simulink model "Crazyflie_NoLinealModel"  (R2020b)
settings: Solver=FixedStepAuto  StartTime=0.0  StopTime=30  FixedStep=0.01  RelTol=1e-3
values from neighbouring files (symbols this model uses):
  fm = 0.2685    [Crazyflie_Model.m]
  g = 9.81    [Crazyflie_Model.m]
  Ixx = 1.395e-05    [Crazyflie_Model.m]
  Iyy = 1.395e-05    [Crazyflie_Model.m]
  Izz = 2.173e-05    [Crazyflie_Model.m]
  m = 0.027    [Crazyflie_Model.m]
  MNL1 = [         CT,           CT,           CT,           CT ... (first row only)    [Crazyflie_Model.m]
  we = sqrt((m*g)/(4*CT))    [Crazyflie_Model.m]
undefined symbols (not defined in the file or in its folder): fs_outer, KDp, KDphi, KDq, KDr, KDtheta, KDxp, KDxv, KDy, KDyaw, KDz, KIp, KIphi, KIq, KIr, KItheta, KIxp, KIxv, KIy, KIyaw, KIz, KPp, KPphi, KPq, KPr, KPtheta, KPxp, KPxv, KPy, KPyaw, KPz, MCO, phi_theta_limit, xyv_lim
libraries: pid_lib x11, simulink x2
settings Model: Creator=Rafael  LastModifiedBy=FranciscoJose
settings DataIOCC: LimitDataPoints=on  SaveFormat=Array  SignalLoggingSaveFormat=ModelDataLogs  ReturnWorkspaceOutputs=off
settings OptimizationCC: ExpressionDepthLimit=2147483647  LifeSpan=inf
settings DebuggingCC: UnderspecifiedInitializationDetection=Classic  MergeDetectMultiDrivingBlocksExec=none  SolverPrmCheckMsg=warning  FcnCallInpInsideContextMsg=warning  AllowSymbolicDim=off  StateNameClashWarn=warning  SFUnexpectedBacktrackingDiag=warning  SFNoUnconditionalDefaultTransitionDiag=warning  SFExecutionAtInitializationDiag=none  ArithmeticOperatorsInVariantConditions=warning
settings HardwareCC: ProdBitPerPointer=32  ProdBitPerSizeT=32  ProdBitPerPtrDiffT=32  ProdLargestAtomicFloat=None  ProdIntDivRoundTo=Undefined  ProdEndianess=Unspecified  ProdWordSize=32  ProdHWDeviceType=32-bit Generic
settings ModelReferenceCC: PropagateSignalLabelsOutOfModel=off
settings SFSimCC: SimUseLocalCustomCode=off  CustomCodeUndefinedFunction=UseInterfaceOnly
settings RTWCC: RTWUseLocalCustomCode=off
settings CodeAppCC: StateflowObjectComments=on
settings GRTTargetCC: TargetLangStandard=C89/C90 (ANSI)
settings ConfigComp: CovMetricSettings=dw  CovSaveCumulativeToWorkspaceVar=on  CovSaveSingleToWorkspaceVar=on  CovExternalEMLEnable=off
settings SimscapeCC: SimscapeNormalizeSystem=off
settings ConfigurationSet: Description=SimMechanics 2G

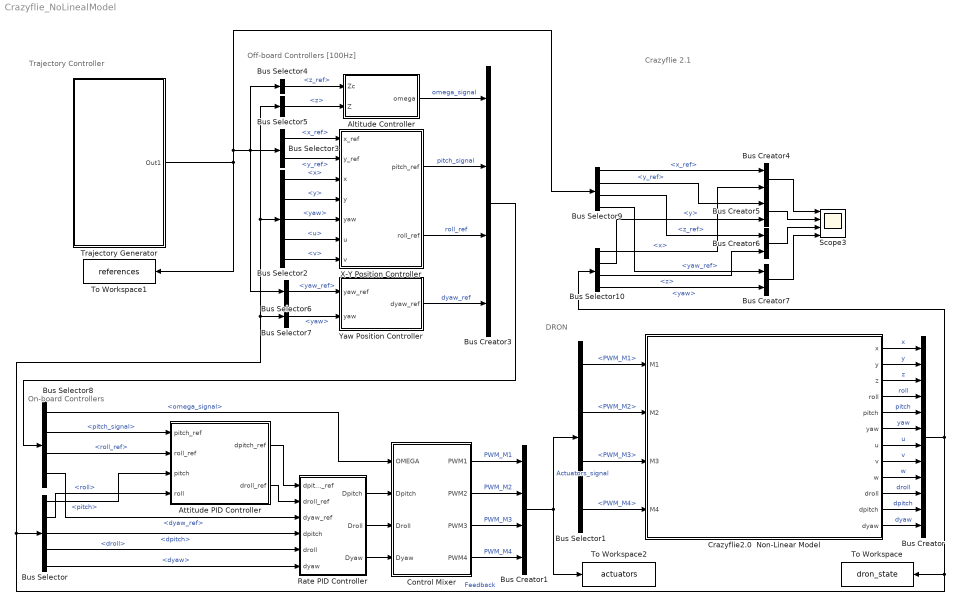
== system Crazyflie_NoLinealModel ==
  note: DRON
  note: Trajectory Controller
  note: Off-board Controllers [100Hz]
  note: On-board Controllers
  note: Crazyflie 2.1
  Altitude Controller : Subsystem
  Attitude PID Controller : Subsystem
  Bus Creator : BusCreator  Inputs=12
  Bus Creator1 : BusCreator  Inputs=4
  Bus Creator3 : BusCreator  Inputs=4
  Bus Creator{4..7} (4 alike) : BusCreator  Inputs=2
  Bus Selector : BusSelector  OutputSignals=pitch,roll,dpitch,droll,dyaw
  Bus Selector1 : BusSelector  OutputSignals=PWM_M1,PWM_M2,PWM_M3,PWM_M4
  Bus Selector10 : BusSelector  OutputSignals=x,y,z,yaw
  Bus Selector2 : BusSelector  OutputSignals=x,y,yaw,u,v
  Bus Selector3 : BusSelector  OutputSignals=x_ref,y_ref
  Bus Selector4 : BusSelector  OutputSignals=z_ref
  Bus Selector5 : BusSelector  OutputSignals=z
  Bus Selector6 : BusSelector  OutputSignals=yaw_ref
  Bus Selector7 : BusSelector  OutputSignals=yaw
  Bus Selector8 : BusSelector  OutputSignals=omega_signal,pitch_signal,roll_ref,dyaw_ref
  Bus Selector9 : BusSelector  OutputSignals=x_ref,y_ref,z_ref,yaw_ref
  Control Mixer : Subsystem
  Crazyflie2.0  Non-Linear Model : Subsystem
      mask Display: image('$imagefile'); % Use "Edit Image" on toolstrip to change.
  Rate PID Controller : Subsystem
  Scope3 : Scope  NumInputPorts=4
  To Workspace : ToWorkspace  VariableName=dron_state  SaveFormat=Timeseries  SampleTime=-1
  To Workspace1 : ToWorkspace  VariableName=references  SaveFormat=Timeseries  SampleTime=-1
  To Workspace2 : ToWorkspace  VariableName=actuators  SaveFormat=Timeseries  SampleTime=-1
  Trajectory Generator : Subsystem
  X-Y Position Controller : Subsystem
  Yaw Position Controller : Subsystem
  wires:
  Crazyflie2.0  Non-Linear Model/11(dpitch) -> Bus Creator/11  "dpitch"
  Crazyflie2.0  Non-Linear Model/3(z) -> Bus Creator/3  "z"
  Crazyflie2.0  Non-Linear Model/12(dyaw) -> Bus Creator/12  "dyaw"
  Crazyflie2.0  Non-Linear Model/4(roll) -> Bus Creator/4  "roll"
  Crazyflie2.0  Non-Linear Model/5(pitch) -> Bus Creator/5  "pitch"
  Crazyflie2.0  Non-Linear Model/6(yaw) -> Bus Creator/6  "yaw"
  Crazyflie2.0  Non-Linear Model/1(x) -> Bus Creator/1  "x"
  Crazyflie2.0  Non-Linear Model/2(y) -> Bus Creator/2  "y"
  Crazyflie2.0  Non-Linear Model/7(u) -> Bus Creator/7  "u"
  Crazyflie2.0  Non-Linear Model/8(v) -> Bus Creator/8  "v"
  Crazyflie2.0  Non-Linear Model/9(w) -> Bus Creator/9  "w"
  Crazyflie2.0  Non-Linear Model/10(droll) -> Bus Creator/10  "droll"
  Bus Creator/1 -> Bus Selector10/1, Bus Selector/1, Bus Selector5/1, Bus Selector2/1, Bus Selector7/1, To Workspace/1  "Feedback"
  Bus Selector/5 -> Rate PID Controller/6(dyaw)  "<dyaw>"
  Control Mixer/1(PWM1) -> Bus Creator1/1  "PWM_M1"
  Control Mixer/2(PWM2) -> Bus Creator1/2  "PWM_M2"
  Control Mixer/3(PWM3) -> Bus Creator1/3  "PWM_M3"
  Control Mixer/4(PWM4) -> Bus Creator1/4  "PWM_M4"
  Bus Creator1/1 -> Bus Selector1/1, To Workspace2/1  "Actuators_signal"
  Bus Selector1/1 -> Crazyflie2.0  Non-Linear Model/1(M1)  "<PWM_M1>"
  Bus Selector1/2 -> Crazyflie2.0  Non-Linear Model/2(M2)  "<PWM_M2>"
  Bus Selector1/3 -> Crazyflie2.0  Non-Linear Model/3(M3)  "<PWM_M3>"
  Bus Selector1/4 -> Crazyflie2.0  Non-Linear Model/4(M4)  "<PWM_M4>"
  Bus Selector4/1 -> Altitude Controller/1(Zc)  "<z_ref>"
  Altitude Controller/1(omega) -> Bus Creator3/1  "omega_signal"
  Bus Selector3/1 -> X-Y Position Controller/1(x_ref)  "<x_ref>"
  Bus Selector3/2 -> X-Y Position Controller/2(y_ref)  "<y_ref>"
  Bus Selector2/1 -> X-Y Position Controller/3(x)  "<x>"
  Bus Selector2/2 -> X-Y Position Controller/4(y)  "<y>"
  Bus Selector2/3 -> X-Y Position Controller/5(yaw)  "<yaw>"
  Bus Selector2/4 -> X-Y Position Controller/6(u)  "<u>"
  Bus Selector2/5 -> X-Y Position Controller/7(v)  "<v>"
  X-Y Position Controller/1(pitch_ref) -> Bus Creator3/2  "pitch_signal"
  X-Y Position Controller/2(roll_ref) -> Bus Creator3/3  "roll_ref"
  Bus Selector5/1 -> Altitude Controller/2(Z)  "<z>"
  Bus Selector6/1 -> Yaw Position Controller/1(yaw_ref)  "<yaw_ref>"
  Bus Selector7/1 -> Yaw Position Controller/2(yaw)  "<yaw>"
  Yaw Position Controller/1(dyaw_ref) -> Bus Creator3/4  "dyaw_ref"
  Bus Creator3/1 -> Bus Selector8/1
  Bus Selector8/1 -> Control Mixer/1(OMEGA)  "<omega_signal>"
  Bus Selector8/2 -> Attitude PID Controller/1(pitch_ref)  "<pitch_signal>"
  Bus Selector8/3 -> Attitude PID Controller/2(roll_ref)  "<roll_ref>"
  Bus Selector8/4 -> Rate PID Controller/3(dyaw_ref)  "<dyaw_ref>"
  Rate PID Controller/1(Dpitch) -> Control Mixer/2(Dpitch)
  Rate PID Controller/3(Dyaw) -> Control Mixer/4(Dyaw)
  Bus Creator4/1 -> Scope3/1
  Bus Creator5/1 -> Scope3/2
  Bus Creator6/1 -> Scope3/3
  Bus Creator7/1 -> Scope3/4
  Bus Selector9/1 -> Bus Creator4/1  "<x_ref>"
  Bus Selector9/2 -> Bus Creator5/1  "<y_ref>"
  Bus Selector9/3 -> Bus Creator6/1  "<z_ref>"
  Bus Selector9/4 -> Bus Creator7/1  "<yaw_ref>"
  Bus Selector10/1 -> Bus Creator4/2  "<x>"
  Bus Selector10/2 -> Bus Creator5/2  "<y>"
  Bus Selector10/3 -> Bus Creator6/2  "<z>"
  Bus Selector10/4 -> Bus Creator7/2  "<yaw>"
  Rate PID Controller/2(Droll) -> Control Mixer/3(Droll)
  Attitude PID Controller/1(dpitch_ref) -> Rate PID Controller/1(dpitch_ref)
  Attitude PID Controller/2(droll_ref) -> Rate PID Controller/2(droll_ref)
  Bus Selector/1 -> Attitude PID Controller/3(pitch)  "<pitch>"
  Bus Selector/2 -> Attitude PID Controller/4(roll)  "<roll>"
  Bus Selector/3 -> Rate PID Controller/4(dpitch)  "<dpitch>"
  Bus Selector/4 -> Rate PID Controller/5(droll)  "<droll>"
  Trajectory Generator/1(Out1) -> To Workspace1/1, Bus Selector9/1, Bus Selector6/1, Bus Selector4/1, Bus Selector3/1

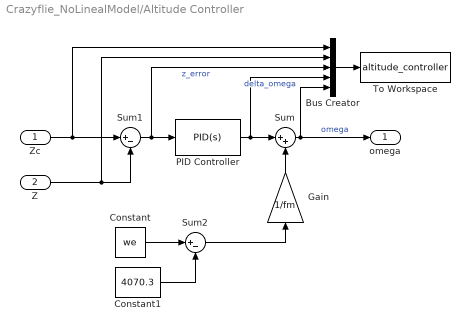
== system Crazyflie_NoLinealModel/Altitude Controller ==
  Zc : Inport
  Z : Inport  Port=2
  Bus Creator : BusCreator  Inputs=5
  Constant : Constant  Value=we
  Constant1 : Constant  Value=4070.3
  Gain : Gain  Gain=1/fm
  PID Controller : pid_lib/PID Controller  Controller=PID  Form=Parallel  TimeDomain=Continuous-time  UseExternalTs=off  SampleTime=-1  IntegratorMethod=Forward Euler  FilterMethod=Forward Euler  ControllerParametersSource=internal  P=KPz  I=KIz  D=KDz  UseFilter=on  N=100  TunerSelectOption=Transfer Function Based (PID Tuner App)  InitialConditionSource=internal  InitialConditionForIntegrator=0  InitialConditionForFilter=0  DifferentiatorICPrevScaledInput=0  ExternalReset=none  TrackingMode=off  Kt=1  LimitOutput=on  SatLimitsSource=internal  UpperSaturationLimit=15000  LowerSaturationLimit=-20000  LinearizeAsGain=on  AntiWindupMode=none  Kb=1/sqrt(KIz)  POutMin=[]  POutMax=[]  IOutMin=[]  IOutMax=[]  DOutMin=[]  DOutMax=[]  NOutMin=[]  NOutMax=[]  SumOutMin=[]  SumOutMax=[]  SaturationOutMin=[]  SaturationOutMax=[]  PParamMin=[]  PParamMax=[]  IParamMin=[]  IParamMax=[]  DParamMin=[]  DParamMax=[]  NParamMin=[]  NParamMax=[]  KbParamMin=[]  KbParamMax=[]  KtParamMin=[]  KtParamMax=[]  KbOutMin=[]  KbOutMax=[]  KtOutMin=[]  KtOutMax=[]  IntegratorOutMin=[]  IntegratorOutMax=[]  FilterOutMin=[]  FilterOutMax=[]  SumI1OutMin=[]  SumI1OutMax=[]  SumI2OutMin=[]  SumI2OutMax=[]  SumI3OutMin=[]  SumI3OutMax=[]  SumI4OutMin=[]  SumI4OutMax=[]  SumDOutMin=[]  SumDOutMax=[]  DifferentiatorOutMin=[]  DifferentiatorOutMax=[]  FilterDiffOutCoefMin=[]  FilterDiffOutCoefMax=[]  ReciprocalOutMin=[]  ReciprocalOutMax=[]  SumDenOutMin=[]  SumDenOutMax=[]  SumNumOutMin=[]  SumNumOutMax=[]  DivideOutMin=[]  DivideOutMax=[]  UdiffTsProdOutMin=[]  UdiffTsProdOutMax=[]  NTsProdOutMin=[]  NTsProdOutMax=[]  UintegralTsProdOutMin=[]  UintegralTsProdOutMax=[]  UngainTsProdOutMin=[]  UngainTsProdOutMax=[]  IntegratorContinuousStateAttributes=''  IntegratorStateMustResolveToSignalObject=off  IntegratorRTWStateStorageClass=Auto  FilterContinuousStateAttributes=''  FilterStateMustResolveToSignalObject=off  FilterRTWStateStorageClass=Auto  ParallelPVariant=InternalParameters  IdealPVariant=Disabled  IVariant=InternalParameters  DVariant=InternalParameters  IntegratorVariant=Continuous  SatVariant=Enabled  AWVariant=Passthrough  PCopyVariant=Disabled  TRVariant=Disabled  FdbkBlocksVariant=Forward  IdealPFdbkVariant=Disabled  SatFdbkVariant=Disabled  DerivativeFilterVariant=ContFilter  NVariant=InternalParameters  NCopyVariant=Disabled  FilterICVariant=InternalICsFilter  IntegratorICVariant=InternalICs  ExternalResetVariant=Disabled  TRSumVariant=Passthrough  SumFdbkVariant=Disabled  SumVariant=Sum_PID  TsampFilterVariant=InternalTs  TsampNgainVariant=Passthrough  TsampIntegralVariant=Passthrough  ExternalSaturationOutDataTypeStr=Inherit: Same as second input
  Sum : Sum  Inputs=|++
  Sum1 : Sum  Inputs=|+-
  Sum2 : Sum  Inputs=|+-
  To Workspace : ToWorkspace  VariableName=altitude_controller  SaveFormat=Timeseries  SampleTime=-1
  omega : Outport
  wires:
  Sum/1 -> Bus Creator/5, omega/1  "omega"
  PID Controller/1 -> Bus Creator/4, Sum/1  "delta_omega"
  Sum1/1 -> Bus Creator/3, PID Controller/1  "z_error"
  Constant/1 -> Sum2/1
  Sum2/1 -> Gain/1
  Constant1/1 -> Sum2/2
  Z/1 -> Sum1/2, Bus Creator/2
  Zc/1 -> Bus Creator/1, Sum1/1
  Gain/1 -> Sum/2
  Bus Creator/1 -> To Workspace/1

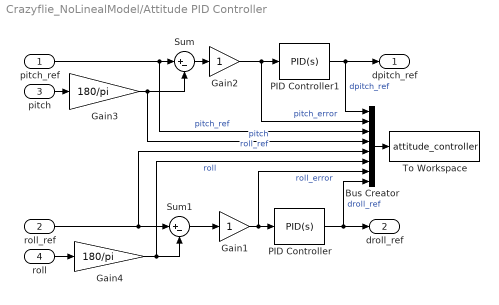
== system Crazyflie_NoLinealModel/Attitude PID Controller ==
  pitch_ref : Inport
  roll_ref : Inport  Port=2
  pitch : Inport  Port=3
  roll : Inport  Port=4
  Bus Creator : BusCreator  Inputs=8
  Gain1 : Gain  SampleTime=1/fs_outer
  Gain2 : Gain  SampleTime=1/fs_outer
  Gain3 : Gain  Gain=180/pi
  Gain4 : Gain  Gain=180/pi
  PID Controller : pid_lib/PID Controller  Controller=PID  Form=Parallel  TimeDomain=Continuous-time  UseExternalTs=off  SampleTime=-1  IntegratorMethod=Forward Euler  FilterMethod=Forward Euler  ControllerParametersSource=internal  P=KPtheta  I=KItheta  D=KDtheta  UseFilter=on  N=100  TunerSelectOption=Transfer Function Based (PID Tuner App)  InitialConditionSource=internal  InitialConditionForIntegrator=0  InitialConditionForFilter=0  DifferentiatorICPrevScaledInput=0  ExternalReset=none  TrackingMode=off  Kt=1  LimitOutput=on  SatLimitsSource=internal  UpperSaturationLimit=phi_theta_limit  LowerSaturationLimit=-phi_theta_limit  LinearizeAsGain=on  AntiWindupMode=back-calculation  Kb=1/sqrt(KItheta)  POutMin=[]  POutMax=[]  IOutMin=[]  IOutMax=[]  DOutMin=[]  DOutMax=[]  NOutMin=[]  NOutMax=[]  SumOutMin=[]  SumOutMax=[]  SaturationOutMin=[]  SaturationOutMax=[]  PParamMin=[]  PParamMax=[]  IParamMin=[]  IParamMax=[]  DParamMin=[]  DParamMax=[]  NParamMin=[]  NParamMax=[]  KbParamMin=[]  KbParamMax=[]  KtParamMin=[]  KtParamMax=[]  KbOutMin=[]  KbOutMax=[]  KtOutMin=[]  KtOutMax=[]  IntegratorOutMin=[]  IntegratorOutMax=[]  FilterOutMin=[]  FilterOutMax=[]  SumI1OutMin=[]  SumI1OutMax=[]  SumI2OutMin=[]  SumI2OutMax=[]  SumI3OutMin=[]  SumI3OutMax=[]  SumI4OutMin=[]  SumI4OutMax=[]  SumDOutMin=[]  SumDOutMax=[]  DifferentiatorOutMin=[]  DifferentiatorOutMax=[]  FilterDiffOutCoefMin=[]  FilterDiffOutCoefMax=[]  ReciprocalOutMin=[]  ReciprocalOutMax=[]  SumDenOutMin=[]  SumDenOutMax=[]  SumNumOutMin=[]  SumNumOutMax=[]  DivideOutMin=[]  DivideOutMax=[]  UdiffTsProdOutMin=[]  UdiffTsProdOutMax=[]  NTsProdOutMin=[]  NTsProdOutMax=[]  UintegralTsProdOutMin=[]  UintegralTsProdOutMax=[]  UngainTsProdOutMin=[]  UngainTsProdOutMax=[]  IntegratorContinuousStateAttributes=''  IntegratorStateMustResolveToSignalObject=off  IntegratorRTWStateStorageClass=Auto  FilterContinuousStateAttributes=''  FilterStateMustResolveToSignalObject=off  FilterRTWStateStorageClass=Auto  ParallelPVariant=InternalParameters  IdealPVariant=Disabled  IVariant=InternalParameters  DVariant=InternalParameters  IntegratorVariant=Continuous  SatVariant=Enabled  AWVariant=BackCalculation  PCopyVariant=Disabled  TRVariant=Disabled  FdbkBlocksVariant=Forward  IdealPFdbkVariant=Disabled  SatFdbkVariant=Disabled  DerivativeFilterVariant=ContFilter  NVariant=InternalParameters  NCopyVariant=Disabled  FilterICVariant=InternalICsFilter  IntegratorICVariant=InternalICs  ExternalResetVariant=Disabled  TRSumVariant=Passthrough  SumFdbkVariant=Disabled  SumVariant=Sum_PID  TsampFilterVariant=InternalTs  TsampNgainVariant=Passthrough  TsampIntegralVariant=Passthrough  ExternalSaturationOutDataTypeStr=Inherit: Same as second input
  PID Controller1 : pid_lib/PID Controller  Controller=PID  Form=Parallel  TimeDomain=Continuous-time  UseExternalTs=off  SampleTime=-1  IntegratorMethod=Forward Euler  FilterMethod=Forward Euler  ControllerParametersSource=internal  P=KPphi  I=KIphi  D=KDphi  UseFilter=on  N=100  TunerSelectOption=Transfer Function Based (PID Tuner App)  InitialConditionSource=internal  InitialConditionForIntegrator=0  InitialConditionForFilter=0  DifferentiatorICPrevScaledInput=0  ExternalReset=none  TrackingMode=off  Kt=1  LimitOutput=on  SatLimitsSource=internal  UpperSaturationLimit=phi_theta_limit  LowerSaturationLimit=-phi_theta_limit  LinearizeAsGain=on  AntiWindupMode=back-calculation  Kb=1/sqrt(KIphi)  POutMin=[]  POutMax=[]  IOutMin=[]  IOutMax=[]  DOutMin=[]  DOutMax=[]  NOutMin=[]  NOutMax=[]  SumOutMin=[]  SumOutMax=[]  SaturationOutMin=[]  SaturationOutMax=[]  PParamMin=[]  PParamMax=[]  IParamMin=[]  IParamMax=[]  DParamMin=[]  DParamMax=[]  NParamMin=[]  NParamMax=[]  KbParamMin=[]  KbParamMax=[]  KtParamMin=[]  KtParamMax=[]  KbOutMin=[]  KbOutMax=[]  KtOutMin=[]  KtOutMax=[]  IntegratorOutMin=[]  IntegratorOutMax=[]  FilterOutMin=[]  FilterOutMax=[]  SumI1OutMin=[]  SumI1OutMax=[]  SumI2OutMin=[]  SumI2OutMax=[]  SumI3OutMin=[]  SumI3OutMax=[]  SumI4OutMin=[]  SumI4OutMax=[]  SumDOutMin=[]  SumDOutMax=[]  DifferentiatorOutMin=[]  DifferentiatorOutMax=[]  FilterDiffOutCoefMin=[]  FilterDiffOutCoefMax=[]  ReciprocalOutMin=[]  ReciprocalOutMax=[]  SumDenOutMin=[]  SumDenOutMax=[]  SumNumOutMin=[]  SumNumOutMax=[]  DivideOutMin=[]  DivideOutMax=[]  UdiffTsProdOutMin=[]  UdiffTsProdOutMax=[]  NTsProdOutMin=[]  NTsProdOutMax=[]  UintegralTsProdOutMin=[]  UintegralTsProdOutMax=[]  UngainTsProdOutMin=[]  UngainTsProdOutMax=[]  IntegratorContinuousStateAttributes=''  IntegratorStateMustResolveToSignalObject=off  IntegratorRTWStateStorageClass=Auto  FilterContinuousStateAttributes=''  FilterStateMustResolveToSignalObject=off  FilterRTWStateStorageClass=Auto  ParallelPVariant=InternalParameters  IdealPVariant=Disabled  IVariant=InternalParameters  DVariant=InternalParameters  IntegratorVariant=Continuous  SatVariant=Enabled  AWVariant=BackCalculation  PCopyVariant=Disabled  TRVariant=Disabled  FdbkBlocksVariant=Forward  IdealPFdbkVariant=Disabled  SatFdbkVariant=Disabled  DerivativeFilterVariant=ContFilter  NVariant=InternalParameters  NCopyVariant=Disabled  FilterICVariant=InternalICsFilter  IntegratorICVariant=InternalICs  ExternalResetVariant=Disabled  TRSumVariant=Passthrough  SumFdbkVariant=Disabled  SumVariant=Sum_PID  TsampFilterVariant=InternalTs  TsampNgainVariant=Passthrough  TsampIntegralVariant=Passthrough  ExternalSaturationOutDataTypeStr=Inherit: Same as second input
  Sum : Sum  Inputs=|+-
  Sum1 : Sum  Inputs=|+-
  To Workspace : ToWorkspace  VariableName=attitude_controller  SaveFormat=Timeseries  SampleTime=-1
  dpitch_ref : Outport
  droll_ref : Outport  Port=2
  wires:
  roll_ref/1 -> Bus Creator/5, Sum1/1  "roll_ref"
  Gain4/1 -> Bus Creator/6, Sum1/2  "roll"
  Gain2/1 -> Bus Creator/2, PID Controller1/1  "pitch_error"
  Sum/1 -> Gain2/1
  pitch_ref/1 -> Bus Creator/3, Sum/1  "pitch_ref"
  Gain3/1 -> Bus Creator/4, Sum/2  "pitch"
  Gain1/1 -> Bus Creator/7, PID Controller/1  "roll_error"
  Sum1/1 -> Gain1/1
  PID Controller/1 -> Bus Creator/8, droll_ref/1  "droll_ref"
  PID Controller1/1 -> Bus Creator/1, dpitch_ref/1  "dpitch_ref"
  pitch/1 -> Gain3/1
  roll/1 -> Gain4/1
  Bus Creator/1 -> To Workspace/1

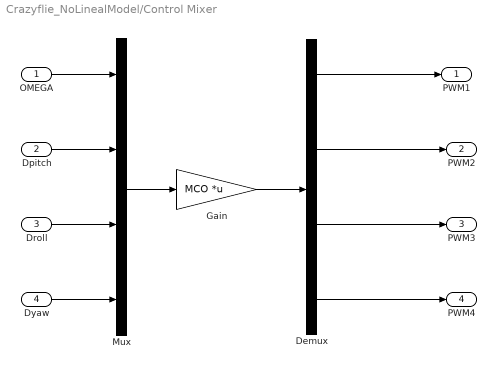
== system Crazyflie_NoLinealModel/Control Mixer ==
  OMEGA : Inport
  Dpitch : Inport  Port=2
  Droll : Inport  Port=3
  Dyaw : Inport  Port=4
  Demux : Demux
  Gain : Gain  Gain=MCO  Multiplication=Matrix(K*u) (u vector)
  Mux : Mux
  PWM1 : Outport
  PWM2 : Outport  Port=2
  PWM3 : Outport  Port=3
  PWM4 : Outport  Port=4
  wires:
  OMEGA/1 -> Mux/1
  Dyaw/1 -> Mux/4
  Demux/4 -> PWM4/1
  Demux/3 -> PWM3/1
  Demux/2 -> PWM2/1
  Demux/1 -> PWM1/1
  Gain/1 -> Demux/1
  Mux/1 -> Gain/1
  Droll/1 -> Mux/3
  Dpitch/1 -> Mux/2

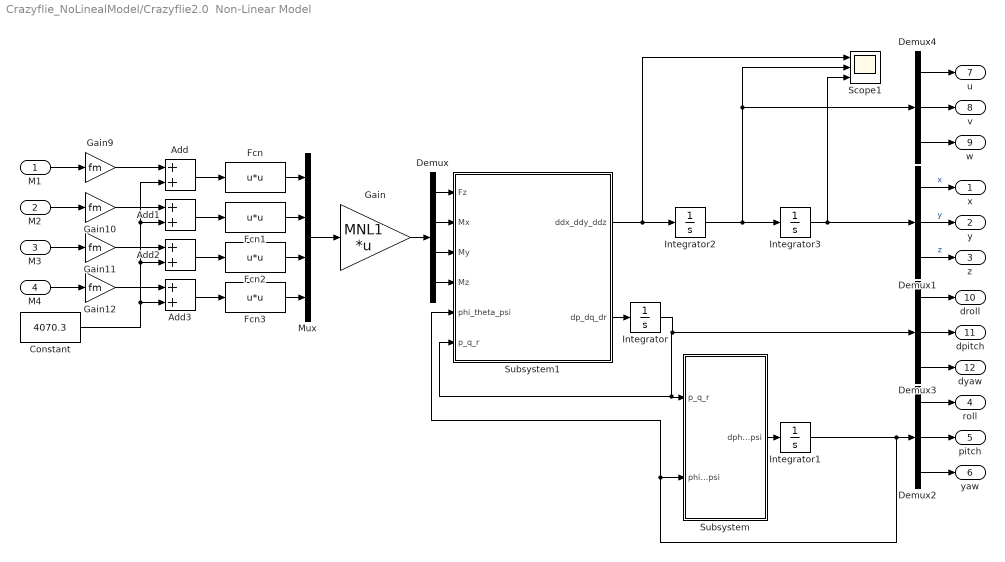
== system Crazyflie_NoLinealModel/Crazyflie2.0  Non-Linear Model ==
  M1 : Inport
  M2 : Inport  Port=2
  M3 : Inport  Port=3
  M4 : Inport  Port=4
  Add{,1..3} (4 alike) : Sum
  Constant : Constant  Value=4070.3
  Demux : Demux
  Demux{1..4} (4 alike) : Demux  Outputs=3
  Fcn{,1..3} (4 alike) : Fcn  Expr=u*u
  Gain : Gain  Gain=MNL1  Multiplication=Matrix(K*u) (u vector)
  Gain{9..12} (4 alike) : Gain  Gain=fm
  Integrator{,1..3} (4 alike) : Integrator
  Mux : Mux
  Scope1 : Scope  NumInputPorts=3
  Subsystem : Subsystem
  Subsystem1 : Subsystem
  x : Outport
  y : Outport  Port=2
  z : Outport  Port=3
  roll : Outport  Port=4
  pitch : Outport  Port=5
  yaw : Outport  Port=6
  u : Outport  Port=7
  v : Outport  Port=8
  w : Outport  Port=9
  droll : Outport  Port=10
  dpitch : Outport  Port=11
  dyaw : Outport  Port=12
  wires:
  Mux/1 -> Gain/1
  Gain/1 -> Demux/1
  Demux/1 -> Subsystem1/1(Fz)
  Demux/2 -> Subsystem1/2(Mx)
  Demux/3 -> Subsystem1/3(My)
  Demux/4 -> Subsystem1/4(Mz)
  Demux1/1 -> x/1  "x"
  Demux1/2 -> y/1  "y"
  Demux1/3 -> z/1  "z"
  Demux2/1 -> roll/1
  Demux2/2 -> pitch/1
  Demux2/3 -> yaw/1
  Demux4/1 -> u/1
  Demux4/2 -> v/1
  Demux4/3 -> w/1
  Demux3/1 -> droll/1
  Demux3/2 -> dpitch/1
  Demux3/3 -> dyaw/1
  M1/1 -> Gain9/1
  M2/1 -> Gain10/1
  M3/1 -> Gain11/1
  M4/1 -> Gain12/1
  Subsystem1/2(dp_dq_dr) -> Integrator/1
  Integrator/1 -> Demux3/1, Subsystem1/6(p_q_r), Subsystem/1(p_q_r)
  Subsystem/1(dphi_dtheta_dpsi) -> Integrator1/1
  Integrator1/1 -> Subsystem1/5(phi_theta_psi), Subsystem/2(phi_theta_psi), Demux2/1
  Subsystem1/1(ddx_ddy_ddz) -> Scope1/1, Integrator2/1
  Integrator2/1 -> Scope1/2, Demux4/1, Integrator3/1
  Integrator3/1 -> Scope1/3, Demux1/1
  Fcn/1 -> Mux/1
  Fcn1/1 -> Mux/2
  Fcn2/1 -> Mux/3
  Fcn3/1 -> Mux/4
  Add/1 -> Fcn/1
  Add1/1 -> Fcn1/1
  Add2/1 -> Fcn2/1
  Add3/1 -> Fcn3/1
  Gain9/1 -> Add/1
  Gain10/1 -> Add1/1
  Gain11/1 -> Add2/1
  Gain12/1 -> Add3/1
  Constant/1 -> Add3/2, Add/2, Add1/2, Add2/2

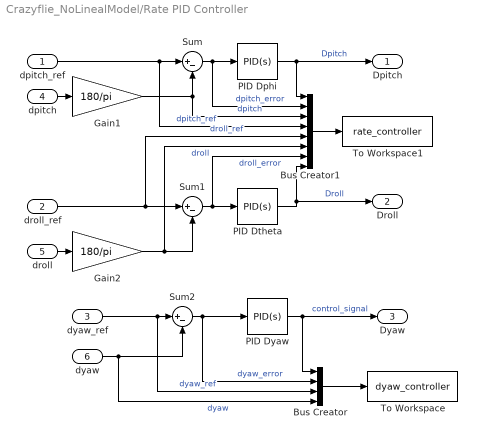
== system Crazyflie_NoLinealModel/Rate PID Controller ==
  dpitch_ref : Inport
  droll_ref : Inport  Port=2
  dyaw_ref : Inport  Port=3
  dpitch : Inport  Port=4
  droll : Inport  Port=5
  dyaw : Inport  Port=6
  Bus Creator : BusCreator  Inputs=4
  Bus Creator1 : BusCreator  Inputs=8
  Gain1 : Gain  Gain=180/pi
  Gain2 : Gain  Gain=180/pi
  PID Dphi : pid_lib/PID Controller  Controller=PID  Form=Parallel  TimeDomain=Continuous-time  UseExternalTs=off  SampleTime=-1  IntegratorMethod=Forward Euler  FilterMethod=Forward Euler  ControllerParametersSource=internal  P=KPp  I=KIp  D=KDp  UseFilter=on  N=100  TunerSelectOption=Transfer Function Based (PID Tuner App)  InitialConditionSource=internal  InitialConditionForIntegrator=0  InitialConditionForFilter=0  DifferentiatorICPrevScaledInput=0  ExternalReset=none  TrackingMode=off  Kt=1  LimitOutput=off  SatLimitsSource=internal  UpperSaturationLimit=inf  LowerSaturationLimit=-inf  LinearizeAsGain=on  AntiWindupMode=none  Kb=1  POutMin=[]  POutMax=[]  IOutMin=[]  IOutMax=[]  DOutMin=[]  DOutMax=[]  NOutMin=[]  NOutMax=[]  SumOutMin=[]  SumOutMax=[]  SaturationOutMin=[]  SaturationOutMax=[]  PParamMin=[]  PParamMax=[]  IParamMin=[]  IParamMax=[]  DParamMin=[]  DParamMax=[]  NParamMin=[]  NParamMax=[]  KbParamMin=[]  KbParamMax=[]  KtParamMin=[]  KtParamMax=[]  KbOutMin=[]  KbOutMax=[]  KtOutMin=[]  KtOutMax=[]  IntegratorOutMin=[]  IntegratorOutMax=[]  FilterOutMin=[]  FilterOutMax=[]  SumI1OutMin=[]  SumI1OutMax=[]  SumI2OutMin=[]  SumI2OutMax=[]  SumI3OutMin=[]  SumI3OutMax=[]  SumI4OutMin=[]  SumI4OutMax=[]  SumDOutMin=[]  SumDOutMax=[]  DifferentiatorOutMin=[]  DifferentiatorOutMax=[]  FilterDiffOutCoefMin=[]  FilterDiffOutCoefMax=[]  ReciprocalOutMin=[]  ReciprocalOutMax=[]  SumDenOutMin=[]  SumDenOutMax=[]  SumNumOutMin=[]  SumNumOutMax=[]  DivideOutMin=[]  DivideOutMax=[]  UdiffTsProdOutMin=[]  UdiffTsProdOutMax=[]  NTsProdOutMin=[]  NTsProdOutMax=[]  UintegralTsProdOutMin=[]  UintegralTsProdOutMax=[]  UngainTsProdOutMin=[]  UngainTsProdOutMax=[]  IntegratorContinuousStateAttributes=''  IntegratorStateMustResolveToSignalObject=off  IntegratorRTWStateStorageClass=Auto  FilterContinuousStateAttributes=''  FilterStateMustResolveToSignalObject=off  FilterRTWStateStorageClass=Auto  ParallelPVariant=InternalParameters  IdealPVariant=Disabled  IVariant=InternalParameters  DVariant=InternalParameters  IntegratorVariant=Continuous  SatVariant=Disabled  AWVariant=Passthrough  PCopyVariant=Disabled  TRVariant=Disabled  FdbkBlocksVariant=Forward  IdealPFdbkVariant=Disabled  SatFdbkVariant=Disabled  DerivativeFilterVariant=ContFilter  NVariant=InternalParameters  NCopyVariant=Disabled  FilterICVariant=InternalICsFilter  IntegratorICVariant=InternalICs  ExternalResetVariant=Disabled  TRSumVariant=Passthrough  SumFdbkVariant=Disabled  SumVariant=Sum_PID  TsampFilterVariant=InternalTs  TsampNgainVariant=Passthrough  TsampIntegralVariant=Passthrough  ExternalSaturationOutDataTypeStr=Inherit: Same as second input
  PID Dtheta : pid_lib/PID Controller  Controller=PID  Form=Parallel  TimeDomain=Continuous-time  UseExternalTs=off  SampleTime=-1  IntegratorMethod=Forward Euler  FilterMethod=Forward Euler  ControllerParametersSource=internal  P=KPq  I=KIq  D=KDq  UseFilter=on  N=100  TunerSelectOption=Transfer Function Based (PID Tuner App)  InitialConditionSource=internal  InitialConditionForIntegrator=0  InitialConditionForFilter=0  DifferentiatorICPrevScaledInput=0  ExternalReset=none  TrackingMode=off  Kt=1  LimitOutput=off  SatLimitsSource=internal  UpperSaturationLimit=inf  LowerSaturationLimit=-inf  LinearizeAsGain=on  AntiWindupMode=none  Kb=1  POutMin=[]  POutMax=[]  IOutMin=[]  IOutMax=[]  DOutMin=[]  DOutMax=[]  NOutMin=[]  NOutMax=[]  SumOutMin=[]  SumOutMax=[]  SaturationOutMin=[]  SaturationOutMax=[]  PParamMin=[]  PParamMax=[]  IParamMin=[]  IParamMax=[]  DParamMin=[]  DParamMax=[]  NParamMin=[]  NParamMax=[]  KbParamMin=[]  KbParamMax=[]  KtParamMin=[]  KtParamMax=[]  KbOutMin=[]  KbOutMax=[]  KtOutMin=[]  KtOutMax=[]  IntegratorOutMin=[]  IntegratorOutMax=[]  FilterOutMin=[]  FilterOutMax=[]  SumI1OutMin=[]  SumI1OutMax=[]  SumI2OutMin=[]  SumI2OutMax=[]  SumI3OutMin=[]  SumI3OutMax=[]  SumI4OutMin=[]  SumI4OutMax=[]  SumDOutMin=[]  SumDOutMax=[]  DifferentiatorOutMin=[]  DifferentiatorOutMax=[]  FilterDiffOutCoefMin=[]  FilterDiffOutCoefMax=[]  ReciprocalOutMin=[]  ReciprocalOutMax=[]  SumDenOutMin=[]  SumDenOutMax=[]  SumNumOutMin=[]  SumNumOutMax=[]  DivideOutMin=[]  DivideOutMax=[]  UdiffTsProdOutMin=[]  UdiffTsProdOutMax=[]  NTsProdOutMin=[]  NTsProdOutMax=[]  UintegralTsProdOutMin=[]  UintegralTsProdOutMax=[]  UngainTsProdOutMin=[]  UngainTsProdOutMax=[]  IntegratorContinuousStateAttributes=''  IntegratorStateMustResolveToSignalObject=off  IntegratorRTWStateStorageClass=Auto  FilterContinuousStateAttributes=''  FilterStateMustResolveToSignalObject=off  FilterRTWStateStorageClass=Auto  ParallelPVariant=InternalParameters  IdealPVariant=Disabled  IVariant=InternalParameters  DVariant=InternalParameters  IntegratorVariant=Continuous  SatVariant=Disabled  AWVariant=Passthrough  PCopyVariant=Disabled  TRVariant=Disabled  FdbkBlocksVariant=Forward  IdealPFdbkVariant=Disabled  SatFdbkVariant=Disabled  DerivativeFilterVariant=ContFilter  NVariant=InternalParameters  NCopyVariant=Disabled  FilterICVariant=InternalICsFilter  IntegratorICVariant=InternalICs  ExternalResetVariant=Disabled  TRSumVariant=Passthrough  SumFdbkVariant=Disabled  SumVariant=Sum_PID  TsampFilterVariant=InternalTs  TsampNgainVariant=Passthrough  TsampIntegralVariant=Passthrough  ExternalSaturationOutDataTypeStr=Inherit: Same as second input
  PID Dyaw : pid_lib/PID Controller  Controller=PID  Form=Parallel  TimeDomain=Continuous-time  UseExternalTs=off  SampleTime=-1  IntegratorMethod=Forward Euler  FilterMethod=Forward Euler  ControllerParametersSource=internal  P=KPr  I=KIr  D=KDr  UseFilter=on  N=100  TunerSelectOption=Transfer Function Based (PID Tuner App)  InitialConditionSource=internal  InitialConditionForIntegrator=0  InitialConditionForFilter=0  DifferentiatorICPrevScaledInput=0  ExternalReset=none  TrackingMode=off  Kt=1  LimitOutput=off  SatLimitsSource=internal  UpperSaturationLimit=inf  LowerSaturationLimit=-inf  LinearizeAsGain=on  AntiWindupMode=none  Kb=1  POutMin=[]  POutMax=[]  IOutMin=[]  IOutMax=[]  DOutMin=[]  DOutMax=[]  NOutMin=[]  NOutMax=[]  SumOutMin=[]  SumOutMax=[]  SaturationOutMin=[]  SaturationOutMax=[]  PParamMin=[]  PParamMax=[]  IParamMin=[]  IParamMax=[]  DParamMin=[]  DParamMax=[]  NParamMin=[]  NParamMax=[]  KbParamMin=[]  KbParamMax=[]  KtParamMin=[]  KtParamMax=[]  KbOutMin=[]  KbOutMax=[]  KtOutMin=[]  KtOutMax=[]  IntegratorOutMin=[]  IntegratorOutMax=[]  FilterOutMin=[]  FilterOutMax=[]  SumI1OutMin=[]  SumI1OutMax=[]  SumI2OutMin=[]  SumI2OutMax=[]  SumI3OutMin=[]  SumI3OutMax=[]  SumI4OutMin=[]  SumI4OutMax=[]  SumDOutMin=[]  SumDOutMax=[]  DifferentiatorOutMin=[]  DifferentiatorOutMax=[]  FilterDiffOutCoefMin=[]  FilterDiffOutCoefMax=[]  ReciprocalOutMin=[]  ReciprocalOutMax=[]  SumDenOutMin=[]  SumDenOutMax=[]  SumNumOutMin=[]  SumNumOutMax=[]  DivideOutMin=[]  DivideOutMax=[]  UdiffTsProdOutMin=[]  UdiffTsProdOutMax=[]  NTsProdOutMin=[]  NTsProdOutMax=[]  UintegralTsProdOutMin=[]  UintegralTsProdOutMax=[]  UngainTsProdOutMin=[]  UngainTsProdOutMax=[]  IntegratorContinuousStateAttributes=''  IntegratorStateMustResolveToSignalObject=off  IntegratorRTWStateStorageClass=Auto  FilterContinuousStateAttributes=''  FilterStateMustResolveToSignalObject=off  FilterRTWStateStorageClass=Auto  ParallelPVariant=InternalParameters  IdealPVariant=Disabled  IVariant=InternalParameters  DVariant=InternalParameters  IntegratorVariant=Continuous  SatVariant=Disabled  AWVariant=Passthrough  PCopyVariant=Disabled  TRVariant=Disabled  FdbkBlocksVariant=Forward  IdealPFdbkVariant=Disabled  SatFdbkVariant=Disabled  DerivativeFilterVariant=ContFilter  NVariant=InternalParameters  NCopyVariant=Disabled  FilterICVariant=InternalICsFilter  IntegratorICVariant=InternalICs  ExternalResetVariant=Disabled  TRSumVariant=Passthrough  SumFdbkVariant=Disabled  SumVariant=Sum_PID  TsampFilterVariant=InternalTs  TsampNgainVariant=Passthrough  TsampIntegralVariant=Passthrough  ExternalSaturationOutDataTypeStr=Inherit: Same as second input
  Sum : Sum  Inputs=|+-
  Sum1 : Sum  Inputs=|+-
  Sum2 : Sum  Inputs=|+-
  To Workspace : ToWorkspace  VariableName=dyaw_controller  SaveFormat=Timeseries  SampleTime=-1
  To Workspace1 : ToWorkspace  VariableName=rate_controller  SaveFormat=Timeseries  SampleTime=-1
  Dpitch : Outport
  Droll : Outport  Port=2
  Dyaw : Outport  Port=3
  wires:
  dpitch_ref/1 -> Bus Creator1/4, Sum/1  "dpitch_ref"
  Gain1/1 -> Bus Creator1/3, Sum/2  "dpitch"
  droll_ref/1 -> Bus Creator1/5, Sum1/1  "droll_ref"
  dyaw_ref/1 -> Bus Creator/3, Sum2/1  "dyaw_ref"
  dyaw/1 -> Bus Creator/4, Sum2/2  "dyaw"
  Sum/1 -> Bus Creator1/2, PID Dphi/1  "dpitch_error"
  PID Dphi/1 -> Bus Creator1/1, Dpitch/1  "Dpitch"
  Sum1/1 -> Bus Creator1/7, PID Dtheta/1  "droll_error"
  PID Dtheta/1 -> Bus Creator1/8, Droll/1  "Droll"
  Sum2/1 -> Bus Creator/2, PID Dyaw/1  "dyaw_error"
  PID Dyaw/1 -> Bus Creator/1, Dyaw/1  "control_signal"
  dpitch/1 -> Gain1/1
  droll/1 -> Gain2/1
  Gain2/1 -> Bus Creator1/6, Sum1/2  "droll"
  Bus Creator/1 -> To Workspace/1
  Bus Creator1/1 -> To Workspace1/1

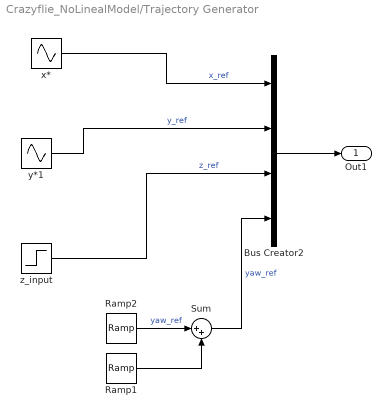
== system Crazyflie_NoLinealModel/Trajectory Generator ==
  Bus Creator2 : BusCreator  Inputs=4
  Ramp1 : simulink/Sources/Ramp  slope=-pi/3  start=10  InitialOutput=0
  Ramp2 : simulink/Sources/Ramp  slope=pi/3  start=0  InitialOutput=0
  Sum : Sum  Inputs=|++
  x* : Sin  Amplitude=0.8  Frequency=2*pi*0.085  Phase=0-0.1  SampleTime=0
  y*1 : Sin  Amplitude=0.8  Frequency=2*pi*0.085  Phase=pi/2-0.1  SampleTime=0
  z_input : Step  Time=0  SampleTime=0
  Out1 : Outport
  wires:
  z_input/1 -> Bus Creator2/3  "z_ref"
  x*/1 -> Bus Creator2/1  "x_ref"
  Ramp1/1 -> Sum/2
  y*1/1 -> Bus Creator2/2  "y_ref"
  Bus Creator2/1 -> Out1/1
  Sum/1 -> Bus Creator2/4  "yaw_ref"
  Ramp2/1 -> Sum/1  "yaw_ref"

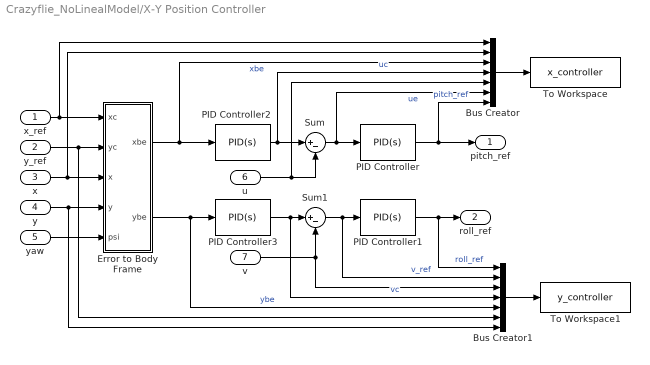
== system Crazyflie_NoLinealModel/X-Y Position Controller ==
  x_ref : Inport
  y_ref : Inport  Port=2
  x : Inport  Port=3
  y : Inport  Port=4
  yaw : Inport  Port=5
  u : Inport  Port=6
  v : Inport  Port=7
  Bus Creator : BusCreator  Inputs=7
  Bus Creator1 : BusCreator  Inputs=7
  Error to Body Frame : MATLAB Function  TreatAsAtomicUnit=on
  PID Controller : pid_lib/PID Controller  Controller=PID  Form=Parallel  TimeDomain=Continuous-time  UseExternalTs=off  SampleTime=-1  IntegratorMethod=Forward Euler  FilterMethod=Forward Euler  ControllerParametersSource=internal  P=KPxv  I=KIxv  D=KDxv  UseFilter=on  N=100  TunerSelectOption=Transfer Function Based (PID Tuner App)  InitialConditionSource=internal  InitialConditionForIntegrator=0  InitialConditionForFilter=0  DifferentiatorICPrevScaledInput=0  ExternalReset=none  TrackingMode=off  Kt=1  LimitOutput=on  SatLimitsSource=internal  UpperSaturationLimit=xyv_lim  LowerSaturationLimit=-xyv_lim  LinearizeAsGain=on  AntiWindupMode=back-calculation  Kb=1/sqrt(2)  POutMin=[]  POutMax=[]  IOutMin=[]  IOutMax=[]  DOutMin=[]  DOutMax=[]  NOutMin=[]  NOutMax=[]  SumOutMin=[]  SumOutMax=[]  SaturationOutMin=[]  SaturationOutMax=[]  PParamMin=[]  PParamMax=[]  IParamMin=[]  IParamMax=[]  DParamMin=[]  DParamMax=[]  NParamMin=[]  NParamMax=[]  KbParamMin=[]  KbParamMax=[]  KtParamMin=[]  KtParamMax=[]  KbOutMin=[]  KbOutMax=[]  KtOutMin=[]  KtOutMax=[]  IntegratorOutMin=[]  IntegratorOutMax=[]  FilterOutMin=[]  FilterOutMax=[]  SumI1OutMin=[]  SumI1OutMax=[]  SumI2OutMin=[]  SumI2OutMax=[]  SumI3OutMin=[]  SumI3OutMax=[]  SumI4OutMin=[]  SumI4OutMax=[]  SumDOutMin=[]  SumDOutMax=[]  DifferentiatorOutMin=[]  DifferentiatorOutMax=[]  FilterDiffOutCoefMin=[]  FilterDiffOutCoefMax=[]  ReciprocalOutMin=[]  ReciprocalOutMax=[]  SumDenOutMin=[]  SumDenOutMax=[]  SumNumOutMin=[]  SumNumOutMax=[]  DivideOutMin=[]  DivideOutMax=[]  UdiffTsProdOutMin=[]  UdiffTsProdOutMax=[]  NTsProdOutMin=[]  NTsProdOutMax=[]  UintegralTsProdOutMin=[]  UintegralTsProdOutMax=[]  UngainTsProdOutMin=[]  UngainTsProdOutMax=[]  IntegratorContinuousStateAttributes=''  IntegratorStateMustResolveToSignalObject=off  IntegratorRTWStateStorageClass=Auto  FilterContinuousStateAttributes=''  FilterStateMustResolveToSignalObject=off  FilterRTWStateStorageClass=Auto  ParallelPVariant=InternalParameters  IdealPVariant=Disabled  IVariant=InternalParameters  DVariant=InternalParameters  IntegratorVariant=Continuous  SatVariant=Enabled  AWVariant=BackCalculation  PCopyVariant=Disabled  TRVariant=Disabled  FdbkBlocksVariant=Forward  IdealPFdbkVariant=Disabled  SatFdbkVariant=Disabled  DerivativeFilterVariant=ContFilter  NVariant=InternalParameters  NCopyVariant=Disabled  FilterICVariant=InternalICsFilter  IntegratorICVariant=InternalICs  ExternalResetVariant=Disabled  TRSumVariant=Passthrough  SumFdbkVariant=Disabled  SumVariant=Sum_PID  TsampFilterVariant=InternalTs  TsampNgainVariant=Passthrough  TsampIntegralVariant=Passthrough  ExternalSaturationOutDataTypeStr=Inherit: Same as second input
  PID Controller1 : pid_lib/PID Controller  Controller=PID  Form=Parallel  TimeDomain=Continuous-time  UseExternalTs=off  SampleTime=-1  IntegratorMethod=Forward Euler  FilterMethod=Forward Euler  ControllerParametersSource=internal  P=KPy  I=KIy  D=KDy  UseFilter=on  N=100  TunerSelectOption=Transfer Function Based (PID Tuner App)  InitialConditionSource=internal  InitialConditionForIntegrator=0  InitialConditionForFilter=0  DifferentiatorICPrevScaledInput=0  ExternalReset=none  TrackingMode=off  Kt=1  LimitOutput=on  SatLimitsSource=internal  UpperSaturationLimit=xyv_lim  LowerSaturationLimit=-xyv_lim  LinearizeAsGain=on  AntiWindupMode=back-calculation  Kb=1/sqrt(2)  POutMin=[]  POutMax=[]  IOutMin=[]  IOutMax=[]  DOutMin=[]  DOutMax=[]  NOutMin=[]  NOutMax=[]  SumOutMin=[]  SumOutMax=[]  SaturationOutMin=[]  SaturationOutMax=[]  PParamMin=[]  PParamMax=[]  IParamMin=[]  IParamMax=[]  DParamMin=[]  DParamMax=[]  NParamMin=[]  NParamMax=[]  KbParamMin=[]  KbParamMax=[]  KtParamMin=[]  KtParamMax=[]  KbOutMin=[]  KbOutMax=[]  KtOutMin=[]  KtOutMax=[]  IntegratorOutMin=[]  IntegratorOutMax=[]  FilterOutMin=[]  FilterOutMax=[]  SumI1OutMin=[]  SumI1OutMax=[]  SumI2OutMin=[]  SumI2OutMax=[]  SumI3OutMin=[]  SumI3OutMax=[]  SumI4OutMin=[]  SumI4OutMax=[]  SumDOutMin=[]  SumDOutMax=[]  DifferentiatorOutMin=[]  DifferentiatorOutMax=[]  FilterDiffOutCoefMin=[]  FilterDiffOutCoefMax=[]  ReciprocalOutMin=[]  ReciprocalOutMax=[]  SumDenOutMin=[]  SumDenOutMax=[]  SumNumOutMin=[]  SumNumOutMax=[]  DivideOutMin=[]  DivideOutMax=[]  UdiffTsProdOutMin=[]  UdiffTsProdOutMax=[]  NTsProdOutMin=[]  NTsProdOutMax=[]  UintegralTsProdOutMin=[]  UintegralTsProdOutMax=[]  UngainTsProdOutMin=[]  UngainTsProdOutMax=[]  IntegratorContinuousStateAttributes=''  IntegratorStateMustResolveToSignalObject=off  IntegratorRTWStateStorageClass=Auto  FilterContinuousStateAttributes=''  FilterStateMustResolveToSignalObject=off  FilterRTWStateStorageClass=Auto  ParallelPVariant=InternalParameters  IdealPVariant=Disabled  IVariant=InternalParameters  DVariant=InternalParameters  IntegratorVariant=Continuous  SatVariant=Enabled  AWVariant=BackCalculation  PCopyVariant=Disabled  TRVariant=Disabled  FdbkBlocksVariant=Forward  IdealPFdbkVariant=Disabled  SatFdbkVariant=Disabled  DerivativeFilterVariant=ContFilter  NVariant=InternalParameters  NCopyVariant=Disabled  FilterICVariant=InternalICsFilter  IntegratorICVariant=InternalICs  ExternalResetVariant=Disabled  TRSumVariant=Passthrough  SumFdbkVariant=Disabled  SumVariant=Sum_PID  TsampFilterVariant=InternalTs  TsampNgainVariant=Passthrough  TsampIntegralVariant=Passthrough  ExternalSaturationOutDataTypeStr=Inherit: Same as second input
  PID Controller2 : pid_lib/PID Controller  Controller=PID  Form=Parallel  TimeDomain=Continuous-time  UseExternalTs=off  SampleTime=-1  IntegratorMethod=Forward Euler  FilterMethod=Forward Euler  ControllerParametersSource=internal  P=KPxp  I=KIxp  D=KDxp  UseFilter=on  N=100  TunerSelectOption=Transfer Function Based (PID Tuner App)  InitialConditionSource=internal  InitialConditionForIntegrator=0  InitialConditionForFilter=0  DifferentiatorICPrevScaledInput=0  ExternalReset=none  TrackingMode=off  Kt=1  LimitOutput=off  SatLimitsSource=internal  UpperSaturationLimit=1.5  LowerSaturationLimit=-1.5  LinearizeAsGain=on  AntiWindupMode=none  Kb=1/sqrt(2)  POutMin=[]  POutMax=[]  IOutMin=[]  IOutMax=[]  DOutMin=[]  DOutMax=[]  NOutMin=[]  NOutMax=[]  SumOutMin=[]  SumOutMax=[]  SaturationOutMin=[]  SaturationOutMax=[]  PParamMin=[]  PParamMax=[]  IParamMin=[]  IParamMax=[]  DParamMin=[]  DParamMax=[]  NParamMin=[]  NParamMax=[]  KbParamMin=[]  KbParamMax=[]  KtParamMin=[]  KtParamMax=[]  KbOutMin=[]  KbOutMax=[]  KtOutMin=[]  KtOutMax=[]  IntegratorOutMin=[]  IntegratorOutMax=[]  FilterOutMin=[]  FilterOutMax=[]  SumI1OutMin=[]  SumI1OutMax=[]  SumI2OutMin=[]  SumI2OutMax=[]  SumI3OutMin=[]  SumI3OutMax=[]  SumI4OutMin=[]  SumI4OutMax=[]  SumDOutMin=[]  SumDOutMax=[]  DifferentiatorOutMin=[]  DifferentiatorOutMax=[]  FilterDiffOutCoefMin=[]  FilterDiffOutCoefMax=[]  ReciprocalOutMin=[]  ReciprocalOutMax=[]  SumDenOutMin=[]  SumDenOutMax=[]  SumNumOutMin=[]  SumNumOutMax=[]  DivideOutMin=[]  DivideOutMax=[]  UdiffTsProdOutMin=[]  UdiffTsProdOutMax=[]  NTsProdOutMin=[]  NTsProdOutMax=[]  UintegralTsProdOutMin=[]  UintegralTsProdOutMax=[]  UngainTsProdOutMin=[]  UngainTsProdOutMax=[]  IntegratorContinuousStateAttributes=''  IntegratorStateMustResolveToSignalObject=off  IntegratorRTWStateStorageClass=Auto  FilterContinuousStateAttributes=''  FilterStateMustResolveToSignalObject=off  FilterRTWStateStorageClass=Auto  ParallelPVariant=InternalParameters  IdealPVariant=Disabled  IVariant=InternalParameters  DVariant=InternalParameters  IntegratorVariant=Continuous  SatVariant=Disabled  AWVariant=Passthrough  PCopyVariant=Disabled  TRVariant=Disabled  FdbkBlocksVariant=Forward  IdealPFdbkVariant=Disabled  SatFdbkVariant=Disabled  DerivativeFilterVariant=ContFilter  NVariant=InternalParameters  NCopyVariant=Disabled  FilterICVariant=InternalICsFilter  IntegratorICVariant=InternalICs  ExternalResetVariant=Disabled  TRSumVariant=Passthrough  SumFdbkVariant=Disabled  SumVariant=Sum_PID  TsampFilterVariant=InternalTs  TsampNgainVariant=Passthrough  TsampIntegralVariant=Passthrough  ExternalSaturationOutDataTypeStr=Inherit: Same as second input
  PID Controller3 : pid_lib/PID Controller  Controller=PID  Form=Parallel  TimeDomain=Continuous-time  UseExternalTs=off  SampleTime=-1  IntegratorMethod=Forward Euler  FilterMethod=Forward Euler  ControllerParametersSource=internal  P=1  I=0  D=0  UseFilter=on  N=100  TunerSelectOption=Transfer Function Based (PID Tuner App)  InitialConditionSource=internal  InitialConditionForIntegrator=0  InitialConditionForFilter=0  DifferentiatorICPrevScaledInput=0  ExternalReset=none  TrackingMode=off  Kt=1  LimitOutput=off  SatLimitsSource=internal  UpperSaturationLimit=1.5  LowerSaturationLimit=-1.5  LinearizeAsGain=on  AntiWindupMode=none  Kb=1/sqrt(2)  POutMin=[]  POutMax=[]  IOutMin=[]  IOutMax=[]  DOutMin=[]  DOutMax=[]  NOutMin=[]  NOutMax=[]  SumOutMin=[]  SumOutMax=[]  SaturationOutMin=[]  SaturationOutMax=[]  PParamMin=[]  PParamMax=[]  IParamMin=[]  IParamMax=[]  DParamMin=[]  DParamMax=[]  NParamMin=[]  NParamMax=[]  KbParamMin=[]  KbParamMax=[]  KtParamMin=[]  KtParamMax=[]  KbOutMin=[]  KbOutMax=[]  KtOutMin=[]  KtOutMax=[]  IntegratorOutMin=[]  IntegratorOutMax=[]  FilterOutMin=[]  FilterOutMax=[]  SumI1OutMin=[]  SumI1OutMax=[]  SumI2OutMin=[]  SumI2OutMax=[]  SumI3OutMin=[]  SumI3OutMax=[]  SumI4OutMin=[]  SumI4OutMax=[]  SumDOutMin=[]  SumDOutMax=[]  DifferentiatorOutMin=[]  DifferentiatorOutMax=[]  FilterDiffOutCoefMin=[]  FilterDiffOutCoefMax=[]  ReciprocalOutMin=[]  ReciprocalOutMax=[]  SumDenOutMin=[]  SumDenOutMax=[]  SumNumOutMin=[]  SumNumOutMax=[]  DivideOutMin=[]  DivideOutMax=[]  UdiffTsProdOutMin=[]  UdiffTsProdOutMax=[]  NTsProdOutMin=[]  NTsProdOutMax=[]  UintegralTsProdOutMin=[]  UintegralTsProdOutMax=[]  UngainTsProdOutMin=[]  UngainTsProdOutMax=[]  IntegratorContinuousStateAttributes=''  IntegratorStateMustResolveToSignalObject=off  IntegratorRTWStateStorageClass=Auto  FilterContinuousStateAttributes=''  FilterStateMustResolveToSignalObject=off  FilterRTWStateStorageClass=Auto  ParallelPVariant=InternalParameters  IdealPVariant=Disabled  IVariant=InternalParameters  DVariant=InternalParameters  IntegratorVariant=Continuous  SatVariant=Disabled  AWVariant=Passthrough  PCopyVariant=Disabled  TRVariant=Disabled  FdbkBlocksVariant=Forward  IdealPFdbkVariant=Disabled  SatFdbkVariant=Disabled  DerivativeFilterVariant=ContFilter  NVariant=InternalParameters  NCopyVariant=Disabled  FilterICVariant=InternalICsFilter  IntegratorICVariant=InternalICs  ExternalResetVariant=Disabled  TRSumVariant=Passthrough  SumFdbkVariant=Disabled  SumVariant=Sum_PID  TsampFilterVariant=InternalTs  TsampNgainVariant=Passthrough  TsampIntegralVariant=Passthrough  ExternalSaturationOutDataTypeStr=Inherit: Same as second input
  Sum : Sum  Inputs=|+-
  Sum1 : Sum  Inputs=|+-
  To Workspace : ToWorkspace  VariableName=x_controller  SaveFormat=Timeseries  SampleTime=-1
  To Workspace1 : ToWorkspace  VariableName=y_controller  SaveFormat=Timeseries  SampleTime=-1
  pitch_ref : Outport
  roll_ref : Outport  Port=2
  wires:
  y/1 -> Bus Creator1/7, Error to Body Frame/4(y)
  x_ref/1 -> Bus Creator/1, Error to Body Frame/1(xc)
  y_ref/1 -> Bus Creator1/6, Error to Body Frame/2(yc)
  x/1 -> Bus Creator/2, Error to Body Frame/3(x)
  v/1 -> Sum1/2, Bus Creator1/3
  u/1 -> Bus Creator/5, Sum/2
  PID Controller2/1 -> Bus Creator/4, Sum/1  "uc"
  PID Controller3/1 -> Bus Creator1/4, Sum1/1  "vc"
  PID Controller/1 -> Bus Creator/7, pitch_ref/1  "pitch_ref"
  Sum/1 -> Bus Creator/6, PID Controller/1  "ue"
  Sum1/1 -> Bus Creator1/2, PID Controller1/1  "v_ref"
  yaw/1 -> Error to Body Frame/5(psi)
  Error to Body Frame/1(xbe) -> Bus Creator/3, PID Controller2/1  "xbe"
  Error to Body Frame/2(ybe) -> Bus Creator1/5, PID Controller3/1  "ybe"
  PID Controller1/1 -> Bus Creator1/1, roll_ref/1  "roll_ref"
  Bus Creator/1 -> To Workspace/1
  Bus Creator1/1 -> To Workspace1/1

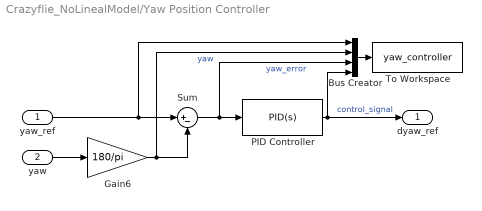
== system Crazyflie_NoLinealModel/Yaw Position Controller ==
  yaw_ref : Inport
  yaw : Inport  Port=2
  Bus Creator : BusCreator  Inputs=4
  Gain6 : Gain  Gain=180/pi
  PID Controller : pid_lib/PID Controller  Controller=PID  Form=Parallel  TimeDomain=Continuous-time  UseExternalTs=off  SampleTime=-1  IntegratorMethod=Forward Euler  FilterMethod=Forward Euler  ControllerParametersSource=internal  P=KPyaw  I=KIyaw  D=KDyaw  UseFilter=on  N=100  TunerSelectOption=Transfer Function Based (PID Tuner App)  InitialConditionSource=internal  InitialConditionForIntegrator=0  InitialConditionForFilter=0  DifferentiatorICPrevScaledInput=0  ExternalReset=none  TrackingMode=off  Kt=1  LimitOutput=on  SatLimitsSource=internal  UpperSaturationLimit=200  LowerSaturationLimit=-200  LinearizeAsGain=on  AntiWindupMode=none  Kb=1  POutMin=[]  POutMax=[]  IOutMin=[]  IOutMax=[]  DOutMin=[]  DOutMax=[]  NOutMin=[]  NOutMax=[]  SumOutMin=[]  SumOutMax=[]  SaturationOutMin=[]  SaturationOutMax=[]  PParamMin=[]  PParamMax=[]  IParamMin=[]  IParamMax=[]  DParamMin=[]  DParamMax=[]  NParamMin=[]  NParamMax=[]  KbParamMin=[]  KbParamMax=[]  KtParamMin=[]  KtParamMax=[]  KbOutMin=[]  KbOutMax=[]  KtOutMin=[]  KtOutMax=[]  IntegratorOutMin=[]  IntegratorOutMax=[]  FilterOutMin=[]  FilterOutMax=[]  SumI1OutMin=[]  SumI1OutMax=[]  SumI2OutMin=[]  SumI2OutMax=[]  SumI3OutMin=[]  SumI3OutMax=[]  SumI4OutMin=[]  SumI4OutMax=[]  SumDOutMin=[]  SumDOutMax=[]  DifferentiatorOutMin=[]  DifferentiatorOutMax=[]  FilterDiffOutCoefMin=[]  FilterDiffOutCoefMax=[]  ReciprocalOutMin=[]  ReciprocalOutMax=[]  SumDenOutMin=[]  SumDenOutMax=[]  SumNumOutMin=[]  SumNumOutMax=[]  DivideOutMin=[]  DivideOutMax=[]  UdiffTsProdOutMin=[]  UdiffTsProdOutMax=[]  NTsProdOutMin=[]  NTsProdOutMax=[]  UintegralTsProdOutMin=[]  UintegralTsProdOutMax=[]  UngainTsProdOutMin=[]  UngainTsProdOutMax=[]  IntegratorContinuousStateAttributes=''  IntegratorStateMustResolveToSignalObject=off  IntegratorRTWStateStorageClass=Auto  FilterContinuousStateAttributes=''  FilterStateMustResolveToSignalObject=off  FilterRTWStateStorageClass=Auto  ParallelPVariant=InternalParameters  IdealPVariant=Disabled  IVariant=InternalParameters  DVariant=InternalParameters  IntegratorVariant=Continuous  SatVariant=Enabled  AWVariant=Passthrough  PCopyVariant=Disabled  TRVariant=Disabled  FdbkBlocksVariant=Forward  IdealPFdbkVariant=Disabled  SatFdbkVariant=Disabled  DerivativeFilterVariant=ContFilter  NVariant=InternalParameters  NCopyVariant=Disabled  FilterICVariant=InternalICsFilter  IntegratorICVariant=InternalICs  ExternalResetVariant=Disabled  TRSumVariant=Passthrough  SumFdbkVariant=Disabled  SumVariant=Sum_PID  TsampFilterVariant=InternalTs  TsampNgainVariant=Passthrough  TsampIntegralVariant=Passthrough  ExternalSaturationOutDataTypeStr=Inherit: Same as second input
  Sum : Sum  Inputs=|+-
  To Workspace : ToWorkspace  VariableName=yaw_controller  SaveFormat=Timeseries  SampleTime=-1
  dyaw_ref : Outport
  wires:
  Sum/1 -> Bus Creator/3, PID Controller/1  "yaw_error"
  Gain6/1 -> Bus Creator/2, Sum/2  "yaw"
  PID Controller/1 -> Bus Creator/4, dyaw_ref/1  "control_signal"
  yaw/1 -> Gain6/1
  yaw_ref/1 -> Bus Creator/1, Sum/1
  Bus Creator/1 -> To Workspace/1

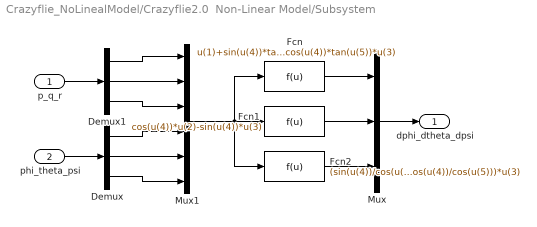
== system Crazyflie_NoLinealModel/Crazyflie2.0  Non-Linear Model/Subsystem ==
  p_q_r : Inport
  phi_theta_psi : Inport  Port=2
  Demux : Demux  Outputs=3
  Demux1 : Demux  Outputs=3
  Fcn : Fcn  Expr=u(1)+sin(u(4))*tan(u(5))*u(2)+cos(u(4))*tan(u(5))*u(3)
  Fcn1 : Fcn  Expr=cos(u(4))*u(2)-sin(u(4))*u(3)
  Fcn2 : Fcn  Expr=(sin(u(4))/cos(u(5)))*u(2)+(cos(u(4))/cos(u(5)))*u(3)
  Mux : Mux  Inputs=3
  Mux1 : Mux  Inputs=6
  dphi_dtheta_dpsi : Outport
  wires:
  Mux1/1 -> Fcn2/1, Fcn/1, Fcn1/1
  Fcn2/1 -> Mux/3
  Fcn/1 -> Mux/1
  Fcn1/1 -> Mux/2
  Mux/1 -> dphi_dtheta_dpsi/1
  Demux/3 -> Mux1/6
  Demux/2 -> Mux1/5
  Demux/1 -> Mux1/4
  Demux1/3 -> Mux1/3
  Demux1/2 -> Mux1/2
  Demux1/1 -> Mux1/1
  phi_theta_psi/1 -> Demux/1
  p_q_r/1 -> Demux1/1

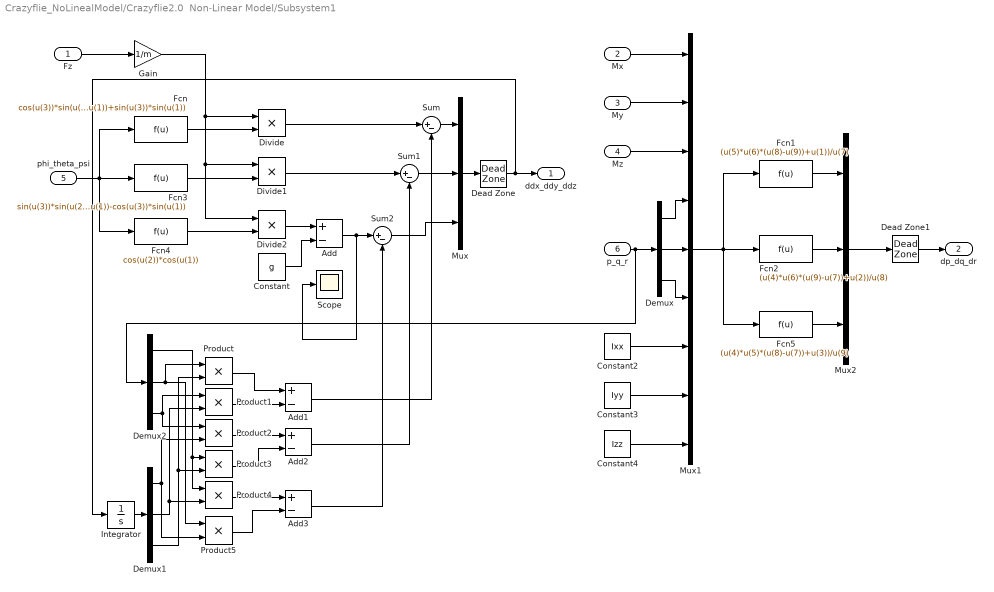
== system Crazyflie_NoLinealModel/Crazyflie2.0  Non-Linear Model/Subsystem1 ==
  Fz : Inport
  Mx : Inport  Port=2
  My : Inport  Port=3
  Mz : Inport  Port=4
  phi_theta_psi : Inport  Port=5
  p_q_r : Inport  Port=6
  Add{,1..3} (4 alike) : Sum  Inputs=+-
  Constant : Constant  Value=g
  Constant2 : Constant  Value=Ixx
  Constant3 : Constant  Value=Iyy
  Constant4 : Constant  Value=Izz
  Dead Zone : DeadZone  LowerValue=-0.0001  UpperValue=0.0001  SaturateOnIntegerOverflow=on
  Dead Zone1 : DeadZone  LowerValue=-0.0001  UpperValue=0.0001  SaturateOnIntegerOverflow=on
  Demux : Demux  Outputs=3
  Demux1 : Demux  Outputs=3
  Demux2 : Demux  Outputs=3
  Divide : Product  Inputs=**
  Divide1 : Product  Inputs=**
  Divide2 : Product  Inputs=**
  Fcn : Fcn  Expr=cos(u(3))*sin(u(2))*cos(u(1))+sin(u(3))*sin(u(1))
  Fcn1 : Fcn  Expr=(u(5)*u(6)*(u(8)-u(9))+u(1))/u(7)
  Fcn2 : Fcn  Expr=(u(4)*u(6)*(u(9)-u(7))+u(2))/u(8)
  Fcn3 : Fcn  Expr=sin(u(3))*sin(u(2))*sin(u(1))-cos(u(3))*sin(u(1))
  Fcn4 : Fcn  Expr=cos(u(2))*cos(u(1))
  Fcn5 : Fcn  Expr=(u(4)*u(5)*(u(8)-u(7))+u(3))/u(9)
  Gain : Gain  Gain=1/m
  Integrator : Integrator
  Mux : Mux  Inputs=3
  Mux1 : Mux  Inputs=9
  Mux2 : Mux  Inputs=3
  Product{,1..5} (6 alike) : Product
  Scope : Scope
  Sum : Sum  Inputs=|+-
  Sum1 : Sum  Inputs=|+-
  Sum2 : Sum  Inputs=|+-
  ddx_ddy_ddz : Outport
  dp_dq_dr : Outport  Port=2
  wires:
  Fz/1 -> Gain/1
  phi_theta_psi/1 -> Fcn/1, Fcn3/1, Fcn4/1
  Fcn/1 -> Divide/2
  Gain/1 -> Divide/1, Divide1/1, Divide2/1
  Fcn3/1 -> Divide1/2
  Fcn4/1 -> Divide2/2
  Divide2/1 -> Add/1
  Constant/1 -> Add/2
  Divide/1 -> Sum/1
  Divide1/1 -> Sum1/1
  Add/1 -> Sum2/1, Scope/1
  p_q_r/1 -> Demux/1, Demux2/1
  Mx/1 -> Mux1/1
  My/1 -> Mux1/2
  Demux/2 -> Mux1/5
  Mz/1 -> Mux1/3
  Demux/1 -> Mux1/4
  Demux/3 -> Mux1/6
  Constant4/1 -> Mux1/9
  Constant3/1 -> Mux1/8
  Constant2/1 -> Mux1/7
  Fcn1/1 -> Mux2/1
  Fcn2/1 -> Mux2/2
  Fcn5/1 -> Mux2/3
  Mux1/1 -> Fcn1/1, Fcn2/1, Fcn5/1
  Mux2/1 -> Dead Zone1/1
  Mux/1 -> Dead Zone/1
  Dead Zone/1 -> ddx_ddy_ddz/1, Integrator/1
  Dead Zone1/1 -> dp_dq_dr/1
  Integrator/1 -> Demux1/1
  Demux2/2 -> Product5/1, Product/1
  Demux1/3 -> Product3/2, Product/2
  Product/1 -> Add1/1
  Demux2/3 -> Product2/1, Product1/1
  Demux1/2 -> Product4/2, Product1/2
  Product1/1 -> Add1/2
  Demux1/1 -> Product5/2, Product2/2
  Product2/1 -> Add2/1
  Demux2/1 -> Product4/1, Product3/1
  Product3/1 -> Add2/2
  Product4/1 -> Add3/1
  Product5/1 -> Add3/2
  Sum/1 -> Mux/1
  Sum1/1 -> Mux/2
  Sum2/1 -> Mux/3
  Add3/1 -> Sum2/2
  Add2/1 -> Sum1/2
  Add1/1 -> Sum/2

== matlab function Crazyflie_NoLinealModel/X-Y Position Controller/Error to Body Frame ==
  data: xc input; xbe output; yc input; x input; y input; psi input; ybe output
function [xbe, ybe] = fcn(xc, yc, x, y, psi)

xe = xc-x;
ye = yc-y;

xbe = xe*cos(psi)+ye*sin(psi);
ybe = -xe*sin(psi)+ye*cos(psi);
